simulink model "furuta3"  (R2017a)
settings: Solver=FixedStepAuto  StartTime=0.0  StopTime=10  FixedStep=dtSim  RelTol=1e-3
values from neighbouring files (symbols this model uses):
  Dp = 5.52e-03    (= 0.00552)    [FurutaSymb3.m]
  Dr = 6.0e-03    (= 0.006)    [FurutaSymb3.m]
  dtDisc = 0.01    [FurutaSymb3.m]
  g = 9.81    [FurutaSymb3.m]    (also in Linear.m)
  J = 0.1    [Linear.m]
  Jp = 0.01    [FurutaSymb3.m]
  Jr = 0.05    [FurutaSymb3.m]
  Jt = Jp*mp*Lr*Lr+Jr*Jp + 0.25 *Jr*mp*Lp*Lp    (= 0.000561822931286)    [FurutaSymb3.m]
  K = place(A,B,[[-0.2+0.2i -0.2-0.2i -0.2]])    [FurutaSymb3.m]    (also in Linear.m = 0.01)
  km = 0.01    [FurutaSymb3.m]
  la = 230.45e-3    (= 0.23045)    [Linear.m]
  lp = 239.73e-3    (= 0.23973)    [Linear.m]
  Lp = 239.73e-3    (= 0.23973)    [FurutaSymb3.m]
  Lr = 230.45e-3    (= 0.23045)    [FurutaSymb3.m]
  M = 0    [Linear.m]    (also in Visualisation.m = scatter3(Xv(2),Yv(2),Zv(2),s,'filled','MarkerFaceColor','b',)
  ma = 0.36233    [Linear.m]
  mp = 0.04948    [FurutaSymb3.m]    (also in Linear.m)
  Rm = 12.38    [FurutaSymb3.m]
  Thetao = 185*pi/180    (= 3.22885911619)    [FurutaSymb3.m]    (also in Linear.m = 0)
undefined symbols (not defined in the file or in its folder): PotMax
settings Model: Creator=felip  LastModifiedBy=felip

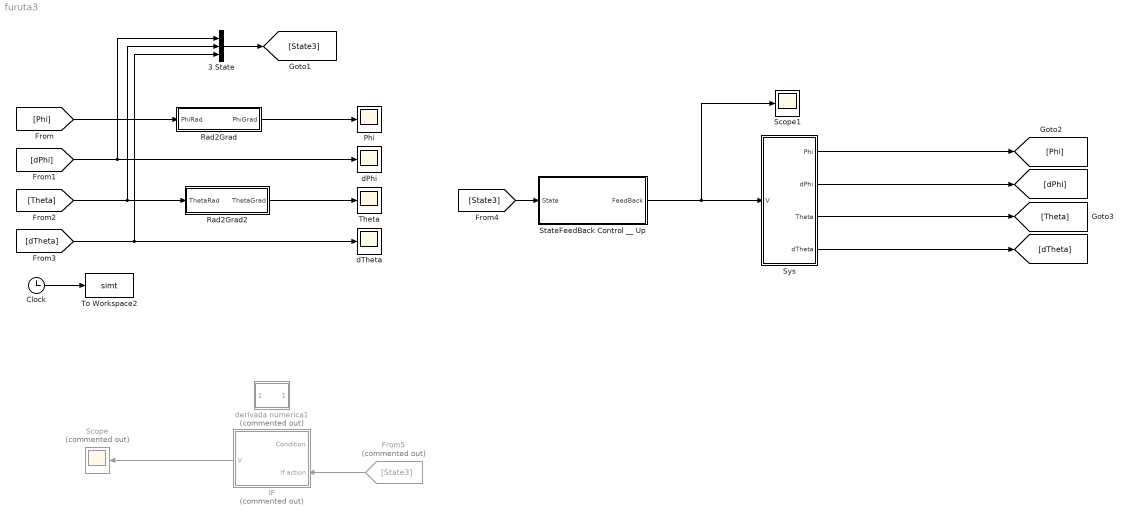
== system furuta3 ==
  3 State : Concatenate  NumInputs=3
  Clock : Clock
  From5 : From  Commented=on  GotoTag=State3
  IF : Subsystem  Commented=on
  Phi : Scope
  Rad2Grad : Subsystem
  Rad2Grad2 : Subsystem
  Scope : Scope  Commented=on
  Scope1 : Scope
  StateFeedBack Control __ Up : Subsystem
  Sys : Subsystem
  Theta : Scope
  To Workspace2 : ToWorkspace  VariableName=simt  SampleTime=-1
      settings: Save2DSignal=2-D array (concatenate along first dimension)
  dPhi : Scope
  dTheta : Scope
  derivada numerica1 : Subsystem  Commented=on
  wires:
  Sys/1(Phi) -> [Phi]
  Sys/2(dPhi) -> [dPhi]
  Sys/4(dTheta) -> [dTheta]
  [Phi] -> Rad2Grad/1(PhiRad)
  [dPhi] -> 3 State/1, dPhi/1
  [Theta] -> 3 State/2, Rad2Grad2/1(ThetaRad)
  [dTheta] -> 3 State/3, dTheta/1
  Rad2Grad/1(PhiGrad) -> Phi/1
  Rad2Grad2/1(ThetaGrad) -> Theta/1
  Clock/1 -> To Workspace2/1
  3 State/1 -> [State3]
  IF/1(V) -> Scope/1
  From5/1 -> IF/2("If action ")
  [State3] -> StateFeedBack Control __ Up/1(State)
  Sys/3(Theta) -> [Theta]
  StateFeedBack Control __ Up/1(FeedBack) -> Scope1/1, Sys/1("V ")

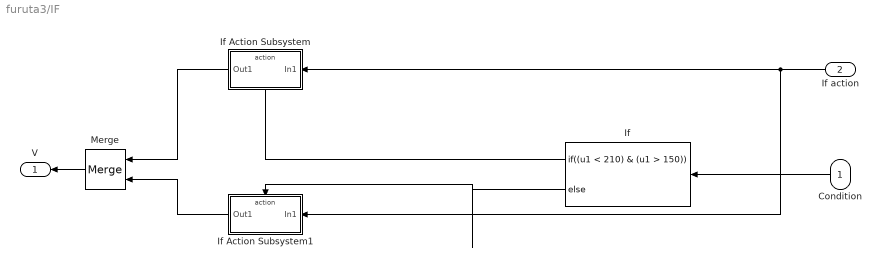
== system furuta3/IF ==
  Condition : Inport
  "If action " : Inport  Port=2
  If : If  IfExpression=(u1 < 210) & (u1 > 150)
  If Action Subsystem : Subsystem  TreatAsAtomicUnit=on
  If Action Subsystem1 : Subsystem  TreatAsAtomicUnit=on
  Merge : Merge
  V : Outport
  wires:
  If/2 -> If Action Subsystem1/Action
  If/1 -> If Action Subsystem/Action
  If Action Subsystem1/1(Out1) -> Merge/2
  "If action "/1 -> If Action Subsystem1/1(In1), If Action Subsystem/1(In1)
  Merge/1 -> V/1
  If Action Subsystem/1(Out1) -> Merge/1
  Condition/1 -> If/1

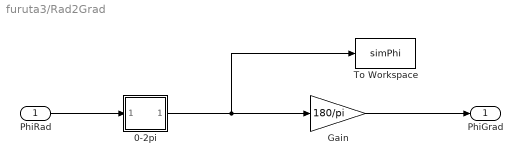
== system furuta3/Rad2Grad ==
  PhiRad : Inport
  0-2pi : Subsystem
  Gain : Gain  Gain=180/pi
  To Workspace : ToWorkspace  VariableName=simPhi  SampleTime=-1
      settings: Save2DSignal=2-D array (concatenate along first dimension)
  PhiGrad : Outport
  wires:
  0-2pi/1(Out1) -> To Workspace/1, Gain/1
  Gain/1 -> PhiGrad/1
  PhiRad/1 -> 0-2pi/1(In1)

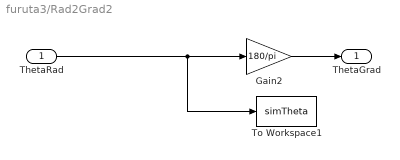
== system furuta3/Rad2Grad2 ==
  ThetaRad : Inport
  Gain2 : Gain  Gain=180/pi
  To Workspace1 : ToWorkspace  VariableName=simTheta  SampleTime=-1
      settings: Save2DSignal=2-D array (concatenate along first dimension)
  ThetaGrad : Outport
  wires:
  Gain2/1 -> ThetaGrad/1
  ThetaRad/1 -> To Workspace1/1, Gain2/1

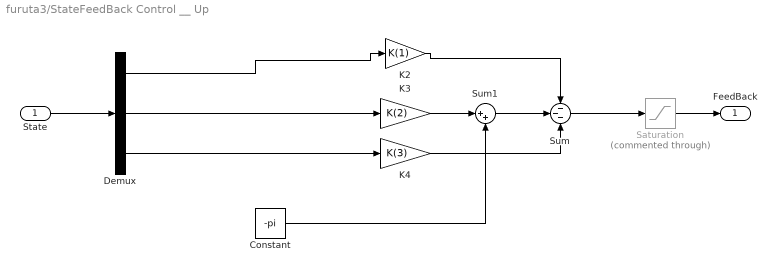
== system furuta3/StateFeedBack Control __ Up ==
  State : Inport
  Constant : Constant  Value=-pi
  Demux : Demux  Outputs=3
  K2 : Gain  Gain=K(1)
  K3 : Gain  Gain=K(2)
  K4 : Gain  Gain=K(3)
  Saturation : Saturate  Commented=through  UpperLimit=12  LowerLimit=-12
  Sum : Sum  Inputs=---
  Sum1 : Sum  Inputs=|++
  FeedBack : Outport
  wires:
  Sum/1 -> Saturation/1
  State/1 -> Demux/1
  Demux/3 -> K4/1
  Saturation/1 -> FeedBack/1
  K2/1 -> Sum/1
  K4/1 -> Sum/3
  Demux/1 -> K2/1
  Demux/2 -> K3/1
  Constant/1 -> Sum1/2
  K3/1 -> Sum1/1
  Sum1/1 -> Sum/2

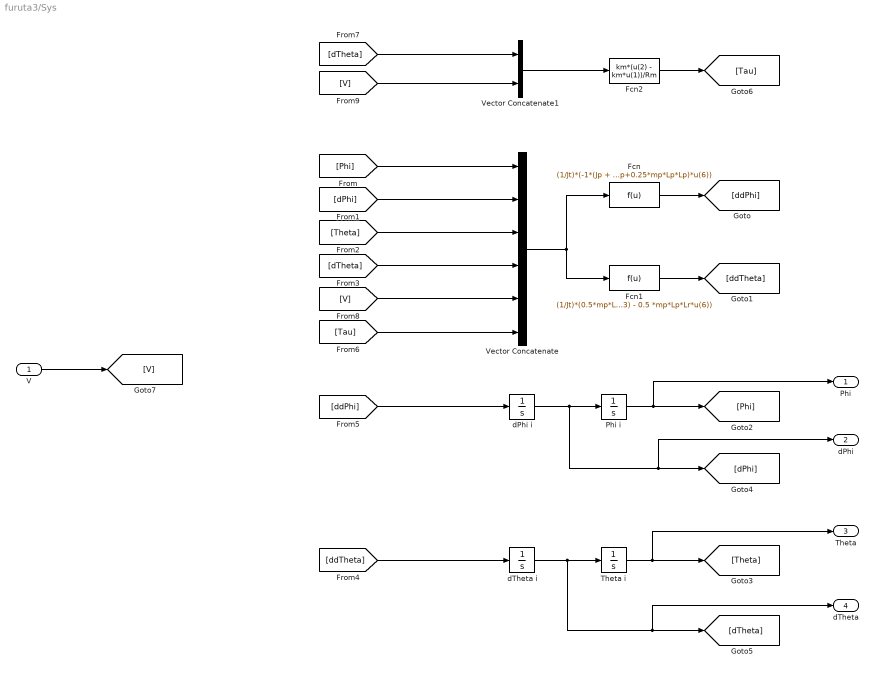
== system furuta3/Sys ==
  "V " : Inport
  Fcn : Fcn  Expr=(1/Jt)*(-1*(Jp + 0.25*mp*Lp*Lp)*Dr*u(2) + 0.5*mp*Lp*Lr*Dp*u(4) + 0.25 *mp*mp*Lp*Lp*g*u(3) + (Jp+0.25*mp*Lp*Lp)*u(6))
  Fcn1 : Fcn  Expr=(1/Jt)*(0.5*mp*Lp*Lr*Dr*u(2) - (Jr + mp*Lr*Lr)*Dp*u(4) - 0.5*mp*Lp*g*(Jr+mp*Lr*Lr)*u(3) - 0.5 *mp*Lp*Lr*u(6))
  Fcn2 : Fcn  Expr=km*(u(2) - km*u(1))/Rm
  Phi i : Integrator
  Theta i : Integrator  InitialCondition=Thetao
  Vector Concatenate : Concatenate  NumInputs=6
  Vector Concatenate1 : Concatenate
  dPhi i : Integrator
  dTheta i : Integrator
  Phi : Outport
  dPhi : Outport  Port=2
  Theta : Outport  Port=3
  dTheta : Outport  Port=4
  wires:
  [Tau] -> Vector Concatenate/6
  [V] -> Vector Concatenate1/2
  Fcn2/1 -> [Tau]
  Vector Concatenate1/1 -> Fcn2/1
  [dTheta] -> Vector Concatenate1/1
  "V "/1 -> [V]
  [dPhi] -> Vector Concatenate/2
  [Theta] -> Vector Concatenate/3
  Vector Concatenate/1 -> Fcn/1, Fcn1/1
  Fcn/1 -> [ddPhi]
  Fcn1/1 -> [ddTheta]
  dPhi i/1 -> dPhi/1, [dPhi], Phi i/1
  Phi i/1 -> Phi/1, [Phi]
  dTheta i/1 -> dTheta/1, [dTheta], Theta i/1
  Theta i/1 -> Theta/1, [Theta]
  [Phi] -> Vector Concatenate/1
  [dTheta] -> Vector Concatenate/4
  [ddPhi] -> dPhi i/1
  [V] -> Vector Concatenate/5
  [ddTheta] -> dTheta i/1

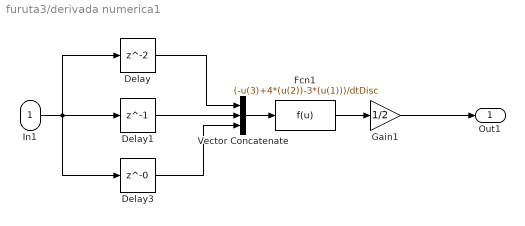
== system furuta3/derivada numerica1 ==
  In1 : Inport
  Delay : Delay  InitialCondition=0  SampleTime=dtDisc
  Delay1 : Delay  DelayLength=1  InitialCondition=0  SampleTime=dtDisc
  Delay3 : Delay  DelayLength=0  InitialCondition=0  SampleTime=dtDisc
  Fcn1 : Fcn  Expr=(-u(3)+4*(u(2))-3*(u(1)))/dtDisc
  Gain1 : Gain  Gain=1/2
  Vector Concatenate : Concatenate  NumInputs=3
  Out1 : Outport
  wires:
  Fcn1/1 -> Gain1/1
  Delay1/1 -> Vector Concatenate/2
  Vector Concatenate/1 -> Fcn1/1
  Delay/1 -> Vector Concatenate/1
  Delay3/1 -> Vector Concatenate/3
  Gain1/1 -> Out1/1
  In1/1 -> Delay1/1, Delay/1, Delay3/1

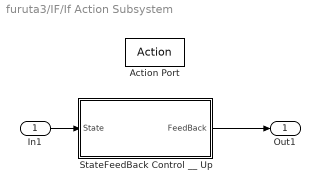
== system furuta3/IF/If Action Subsystem ==
  In1 : Inport
  Action Port : ActionPort  ActionType=then
  StateFeedBack Control __ Up : Subsystem
  Out1 : Outport
  wires:
  In1/1 -> StateFeedBack Control __ Up/1(State)
  StateFeedBack Control __ Up/1(FeedBack) -> Out1/1

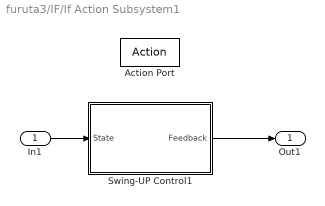
== system furuta3/IF/If Action Subsystem1 ==
  In1 : Inport
  Action Port : ActionPort  ActionType=else
  Swing-UP Control1 : Subsystem
  Out1 : Outport  InitialOutput=0
  wires:
  Swing-UP Control1/1(Feedback) -> Out1/1
  In1/1 -> Swing-UP Control1/1(State)

== system furuta3/Rad2Grad/0-2pi ==
  In1 : Inport
  2pi : Constant  Value=2*pi
  Math Function : Math  Operator=mod  SaturateOnIntegerOverflow=on
  Out1 : Outport
  wires:
  2pi/1 -> Math Function/2
  Math Function/1 -> Out1/1
  In1/1 -> Math Function/1

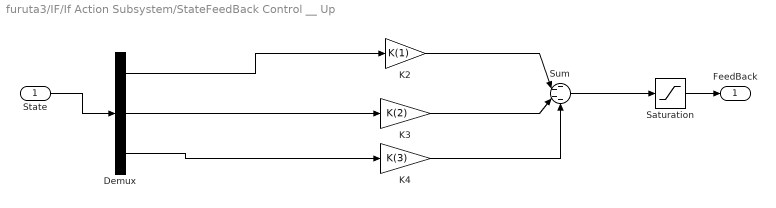
== system furuta3/IF/If Action Subsystem/StateFeedBack Control __ Up ==
  State : Inport
  Demux : Demux  Outputs=3
  K2 : Gain  Gain=K(1)
  K3 : Gain  Gain=K(2)
  K4 : Gain  Gain=K(3)
  Saturation : Saturate  UpperLimit=12  LowerLimit=-12
  Sum : Sum  Inputs=----
  FeedBack : Outport
  wires:
  Demux/2 -> K3/1
  Sum/1 -> Saturation/1
  State/1 -> Demux/1
  Demux/3 -> K4/1
  Saturation/1 -> FeedBack/1
  K2/1 -> Sum/2
  K3/1 -> Sum/3
  K4/1 -> Sum/4
  Demux/1 -> K2/1

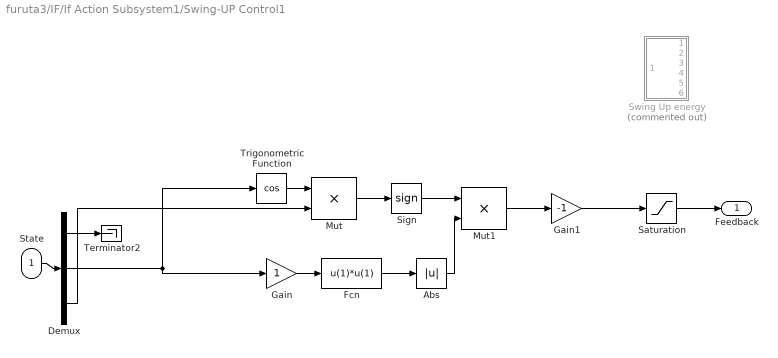
== system furuta3/IF/If Action Subsystem1/Swing-UP Control1 ==
  State : Inport
  Abs : Abs
  Demux : Demux  Outputs=3
  Fcn : Fcn  Expr=u(1)*u(1)
  Gain : Gain
  Gain1 : Gain  Gain=-1
  Mut : Product  Inputs=**
  Mut1 : Product  Inputs=**
  Saturation : Saturate  UpperLimit=12  LowerLimit=-12
  Sign : Signum
  Swing Up energy : Subsystem  Commented=on
  Terminator2 : Terminator
  Trigonometric Function : Trigonometry  Operator=cos
  Feedback : Outport
  wires:
  Saturation/1 -> Feedback/1
  State/1 -> Demux/1
  Gain/1 -> Fcn/1
  Mut/1 -> Sign/1
  Sign/1 -> Mut1/1
  Abs/1 -> Mut1/2
  Demux/3 -> Mut/2
  Trigonometric Function/1 -> Mut/1
  Fcn/1 -> Abs/1
  Demux/2 -> Trigonometric Function/1, Gain/1
  Mut1/1 -> Gain1/1
  Gain1/1 -> Saturation/1
  Demux/1 -> Terminator2/1

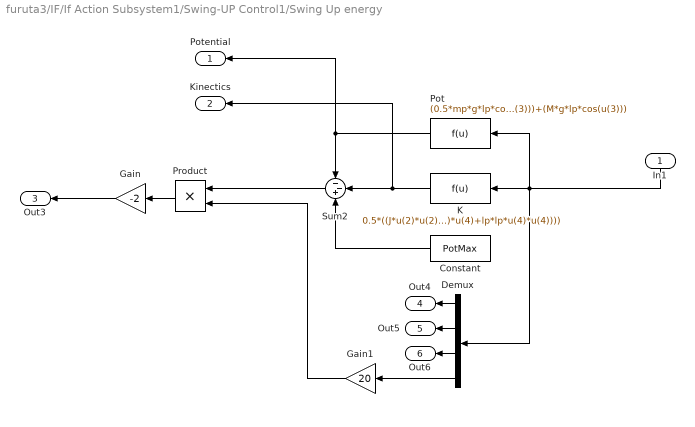
== system furuta3/IF/If Action Subsystem1/Swing-UP Control1/Swing Up energy ==
  In1 : Inport
  Constant : Constant  Value=PotMax
  Demux : Demux
  Gain : Gain  Gain=-2
  Gain1 : Gain  Gain=20
  K : Fcn  Expr=0.5*((J*u(2)*u(2))+(ma*la*la*u(2)*u(2)/3)+(mp*(la*la+lp*lp*sin(u(3))*sin(u(3))/3)*u(2)*u(2))+(mp*la*lp*cos(u(3))*u(2)*u(4))+(mp*lp*lp*u(4)*u(4)/3)+(M*((la*la+lp*lp*sin(u(3))*sin(u(3)))*u(2)*u(2)+2*la*lp*cos(u(3))*u(2)*u(4)+lp*lp*u(4)*u(4))))
  Pot : Fcn  Expr=(0.5*mp*g*lp*cos(u(3)))+(M*g*lp*cos(u(3)))
  Product : Product
  Sum2 : Sum  Inputs=--+
  Potential : Outport
  Kinectics : Outport  Port=2
  Out3 : Outport  Port=3
  Out4 : Outport  Port=4
  Out5 : Outport  Port=5
  Out6 : Outport  Port=6
  wires:
  Demux/3 -> Out6/1
  Demux/2 -> Out5/1
  Demux/1 -> Out4/1
  Pot/1 -> Potential/1, Sum2/1
  Constant/1 -> Sum2/3
  K/1 -> Kinectics/1, Sum2/2
  Gain/1 -> Out3/1
  Gain1/1 -> Product/2
  In1/1 -> Demux/1, Pot/1, K/1
  Sum2/1 -> Product/1
  Demux/4 -> Gain1/1
  Product/1 -> Gain/1
